simulink model "fxpdemo_direct_form2"  (Simulink 5.0)
settings: Solver=FixedStepDiscrete  SolverMode=SingleTasking  StartTime=0.0  StopTime=200.0  FixedStep=1  RelTol=1e-3
libraries: fixpt_lib_4 x2
settings Model: CovMetricSettings=d  MinMaxOverflowLogging=MinMaxAndOverflow  Creator=andyb  LastModifiedBy=andyb  ExtModeTrigMode=oneshot  ExtModeArmWhenConnect=off  ExtModeAutoUpdateStatusClock=off  LimitDataPoints=off  IntegerOverflowMsg=none  ParameterDowncastMsg=warning  ParameterOverflowMsg=warning  ParameterPrecisionLossMsg=none  BooleanDataType=off  RTWOptions="-aRollThreshold=5 -aShowEliminatedStatements=1 -aRTWVerbose=1 -aLocalBlockOutputs=1 -aInlineInvariantSignals=1 -aLogVarNameModifier=\"rt_\" -aExtMode=0"

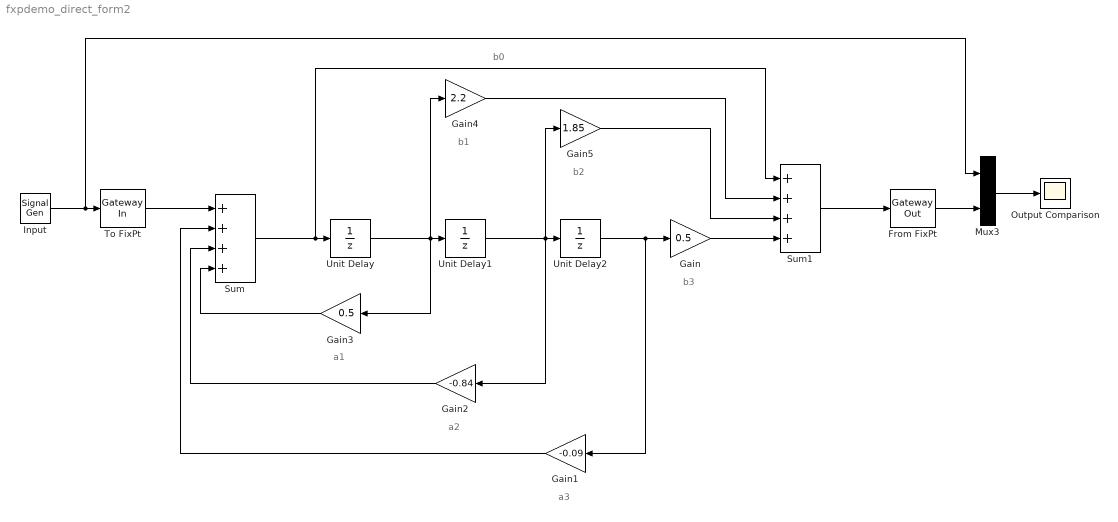
== system fxpdemo_direct_form2 ==
  note: b0
  note: b1
  note: b2
  note: b3
  note: a1
  note: a2
  note: a3
  From FixPt : fixpt_lib_4/Data Type/Gateway Out  OutRealWorld=Real World Value  OutBuiltInType=double  DoSatur=off
  Gain : Gain  Gain=0.5  ShowAdditionalParam=on  ParameterDataTypeMode=Specify via dialog  ParameterDataType=sfix( 16 )  ParameterScalingMode=Best Precision: Column-wise  ParameterScaling=2^-10  OutDataTypeMode=Specify via dialog  OutScaling=2^-10
  Gain1 : Gain  Orientation=left  Gain=-0.09  ShowAdditionalParam=on  ParameterDataTypeMode=Specify via dialog  ParameterDataType=sfix( 16 )  ParameterScalingMode=Best Precision: Column-wise  ParameterScaling=2^-10  OutDataTypeMode=Specify via dialog  OutScaling=2^-10
  Gain2 : Gain  Orientation=left  Gain=-0.84  ShowAdditionalParam=on  ParameterDataTypeMode=Specify via dialog  ParameterDataType=sfix( 16 )  ParameterScalingMode=Best Precision: Column-wise  ParameterScaling=2^-10  OutDataTypeMode=Specify via dialog  OutScaling=2^-10
  Gain3 : Gain  Orientation=left  Gain=0.5  ShowAdditionalParam=on  ParameterDataTypeMode=Specify via dialog  ParameterDataType=sfix( 16 )  ParameterScalingMode=Best Precision: Column-wise  ParameterScaling=2^-10  OutDataTypeMode=Specify via dialog  OutScaling=2^-10
  Gain4 : Gain  Gain=2.2  ShowAdditionalParam=on  ParameterDataTypeMode=Specify via dialog  ParameterDataType=sfix( 16 )  ParameterScalingMode=Best Precision: Column-wise  ParameterScaling=2^-10  OutDataTypeMode=Specify via dialog  OutScaling=2^-10
  Gain5 : Gain  Gain=1.85  ShowAdditionalParam=on  ParameterDataTypeMode=Specify via dialog  ParameterDataType=sfix( 16 )  ParameterScalingMode=Best Precision: Column-wise  ParameterScaling=2^-10  OutDataTypeMode=Specify via dialog  OutScaling=2^-10
  Input : SignalGenerator  WaveForm=square  Frequency=0.005
  Mux3 : Mux  Inputs=2
  Output Comparison : Scope
      settings: TickLabels=on  TimeRange=200  YMin=-8  YMax=10  SaveName=OutputComparison
  Sum : Sum  Inputs=++++  ShowAdditionalParam=on  OutDataTypeMode=Specify via dialog  OutScaling=2^-10
  Sum1 : Sum  Inputs=++++  ShowAdditionalParam=on  OutDataTypeMode=Specify via dialog  OutScaling=2^-10
  To FixPt : fixpt_lib_4/Data Type/Gateway In  InRealWorld=Real World Value  OutputDataTypeScalingMode=Specify via dialog  OutDataType=sfix(16)  OutScaling=2^-10  DoSatur=off
  Unit Delay : UnitDelay  X0=0.0  SampleTime=1.0
  Unit Delay1 : UnitDelay  X0=0.0  SampleTime=1.0
  Unit Delay2 : UnitDelay  X0=0.0  SampleTime=1.0
  wires:
  Input/1 -> To FixPt/1, Mux3/1
  To FixPt/1 -> Sum/1
  Sum/1 -> Unit Delay/1, Sum1/1
  Gain3/1 -> Sum/4
  Unit Delay/1 -> Unit Delay1/1, Gain3/1, Gain4/1
  Gain2/1 -> Sum/3
  Unit Delay1/1 -> Unit Delay2/1, Gain2/1, Gain5/1
  Gain1/1 -> Sum/2
  Gain/1 -> Sum1/4
  Gain5/1 -> Sum1/3
  Gain4/1 -> Sum1/2
  Unit Delay2/1 -> Gain/1, Gain1/1
  Sum1/1 -> From FixPt/1
  From FixPt/1 -> Mux3/2
  Mux3/1 -> Output Comparison/1
